simulink model "blockdemo"  (Simulink 6.3)
settings: Solver=VariableStepDiscrete  StartTime=0  StopTime=20  RelTol=1e-3
InitFcn:
  | %% DSPBuilder Start
  | alt_dspbuilder_update_model(bdroot)
  | %% DSPBuilder End
libraries: allblocks_alteradspbuilder2 x12
settings Model: Creator=mjervis  LastModifiedBy=delphick
settings DataIOCC: SignalLoggingName=sigsOut
settings OptimizationCC: BlockReduction=off  BooleanDataType=off  InlineInvariantSignals=on
settings DebuggingCC: SolverPrmCheckMsg=none
settings HardwareCC: TargetUnknown=on

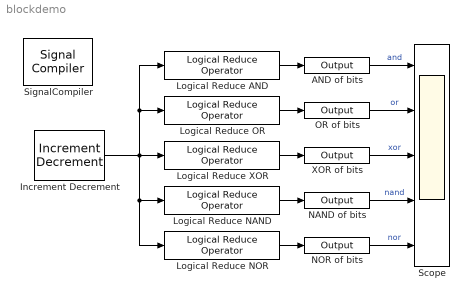
== system blockdemo ==
  AND of bits : allblocks_alteradspbuilder2/Output  iofile=C:\workspace_clean\Documentation\DesignExamples\Tutorials\UnitBlocks\GateAndControl\LogicalReduceOperator\tb_blockdemo\blockdemo_AND+of+bits.capture  BusType=Single Bit  bwl=8  bwr=0  PORTTYPE=Output
  Increment Decrement : allblocks_alteradspbuilder2/Increment Decrement  BusType=Unsigned Integer  bwl=4  bwr=8  SpecifyClock=off  clr_value=0  direction=Increment  phase_selection=1  use_ena=off  use_sclr=off
      settings: AttributesFormatString=%<BusType>
  Logical Reduce AND : allblocks_alteradspbuilder2/Logical Reduce Operator  BusType=Unsigned Integer  bwl=4  bwr=0  LogicalOperator=AND
  Logical Reduce NAND : allblocks_alteradspbuilder2/Logical Reduce Operator  BusType=Unsigned Integer  bwl=4  bwr=0  LogicalOperator=NAND
  Logical Reduce NOR : allblocks_alteradspbuilder2/Logical Reduce Operator  BusType=Unsigned Integer  bwl=4  bwr=0  LogicalOperator=NOR
  Logical Reduce OR : allblocks_alteradspbuilder2/Logical Reduce Operator  BusType=Unsigned Integer  bwl=4  bwr=0  LogicalOperator=OR
  Logical Reduce XOR : allblocks_alteradspbuilder2/Logical Reduce Operator  BusType=Unsigned Integer  bwl=4  bwr=0  LogicalOperator=XOR
  NAND of bits : allblocks_alteradspbuilder2/Output  iofile=C:\workspace_clean\Documentation\DesignExamples\Tutorials\UnitBlocks\GateAndControl\LogicalReduceOperator\tb_blockdemo\blockdemo_NAND+of+bits.capture  BusType=Single Bit  bwl=8  bwr=0  PORTTYPE=Output
  NOR of bits : allblocks_alteradspbuilder2/Output  iofile=C:\workspace_clean\Documentation\DesignExamples\Tutorials\UnitBlocks\GateAndControl\LogicalReduceOperator\tb_blockdemo\blockdemo_NOR+of+bits.capture  BusType=Single Bit  bwl=8  bwr=0  PORTTYPE=Output
  OR of bits : allblocks_alteradspbuilder2/Output  iofile=C:\workspace_clean\Documentation\DesignExamples\Tutorials\UnitBlocks\GateAndControl\LogicalReduceOperator\tb_blockdemo\blockdemo_OR+of+bits.capture  BusType=Single Bit  bwl=8  bwr=0  PORTTYPE=Output
  Scope : Scope  NumInputPorts=5
      settings: YMin=-1~-1~-1~-1~-1  YMax=2~2~2~2~2  SampleInput=on  SampleTime=1
  SignalCompiler : allblocks_alteradspbuilder2/Signal Compiler  DeviceFamily=Stratix IV  DeviceName=AUTO  EnableSignalTap=off  SignalTapDepth=128  UseBoardBlock=off  StpUseDefaultClock=on  StpClock=clock
  XOR of bits : allblocks_alteradspbuilder2/Output  iofile=C:\workspace_clean\Documentation\DesignExamples\Tutorials\UnitBlocks\GateAndControl\LogicalReduceOperator\tb_blockdemo\blockdemo_XOR+of+bits.capture  BusType=Single Bit  bwl=8  bwr=0  PORTTYPE=Output
  wires:
  AND of bits/1 -> Scope/1  "and"
  OR of bits/1 -> Scope/2  "or"
  XOR of bits/1 -> Scope/3  "xor"
  Increment Decrement/1 -> Logical Reduce AND/1, Logical Reduce OR/1, Logical Reduce XOR/1, Logical Reduce NOR/1, Logical Reduce NAND/1
  NAND of bits/1 -> Scope/4  "nand"
  NOR of bits/1 -> Scope/5  "nor"
  Logical Reduce AND/1 -> AND of bits/1
  Logical Reduce OR/1 -> OR of bits/1
  Logical Reduce XOR/1 -> XOR of bits/1
  Logical Reduce NAND/1 -> NAND of bits/1
  Logical Reduce NOR/1 -> NOR of bits/1
